simulink model "Problem6"  (R2021a)
settings: Solver=VariableStepAuto  StartTime=0.0  StopTime=10.0  RelTol=1e-3
settings Model: Creator=Nida  LastModifiedBy=Nida

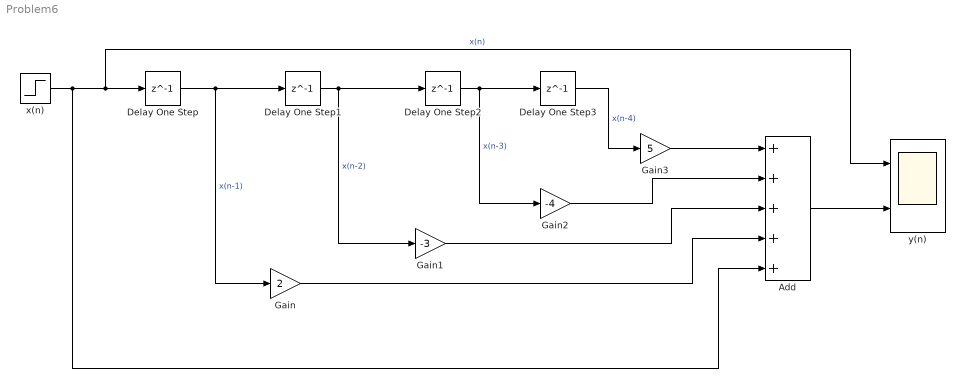
== system Problem6 ==
  Add : Sum  Inputs=+++++
  Delay One Step{,1..3} (4 alike) : Delay  DelayLength=1
  Gain : Gain  Gain=2
  Gain1 : Gain  Gain=-3
  Gain2 : Gain  Gain=-4
  Gain3 : Gain  Gain=5
  x(n) : Step  SampleTime=0
  y(n) : Scope  NumInputPorts=2
  wires:
  Delay One Step/1 -> Gain/1, Delay One Step1/1  "x(n-1)"
  Delay One Step1/1 -> Gain1/1, Delay One Step2/1  "x(n-2)"
  Delay One Step2/1 -> Gain2/1, Delay One Step3/1  "x(n-3)"
  Delay One Step3/1 -> Gain3/1  "x(n-4)"
  Gain3/1 -> Add/1
  Gain2/1 -> Add/2
  Gain1/1 -> Add/3
  Gain/1 -> Add/4
  x(n)/1 -> Add/5, y(n)/1, Delay One Step/1  "x(n)"
  Add/1 -> y(n)/2
